simulink model "theirs"  (R2018b)
settings: Solver=VariableStepAuto  StartTime=0.0  StopTime=10.0  RelTol=1e-3
settings Model: Creator=rjongeli  LastModifiedBy=rjongeli

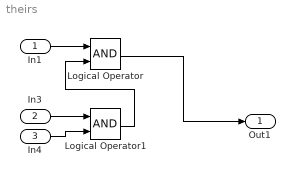
== system theirs ==
  In1 : Inport
  In3 : Inport  Port=2
  In4 : Inport  Port=3
  Logical Operator : Logic  AllPortsSameDT=off  OutDataTypeStr=boolean
  Logical Operator1 : Logic  AllPortsSameDT=off  OutDataTypeStr=boolean
  Out1 : Outport
  wires:
  In1/1 -> Logical Operator/1
  In3/1 -> Logical Operator1/1
  In4/1 -> Logical Operator1/2
  Logical Operator/1 -> Out1/1
  Logical Operator1/1 -> Logical Operator/2
